simulink model "final_test"  (R2017a)
settings: Solver=VariableStepAuto  StartTime=0.0  StopTime=10.0  RelTol=1e-3
settings Model: Creator=ashwi  LastModifiedBy=ashwi

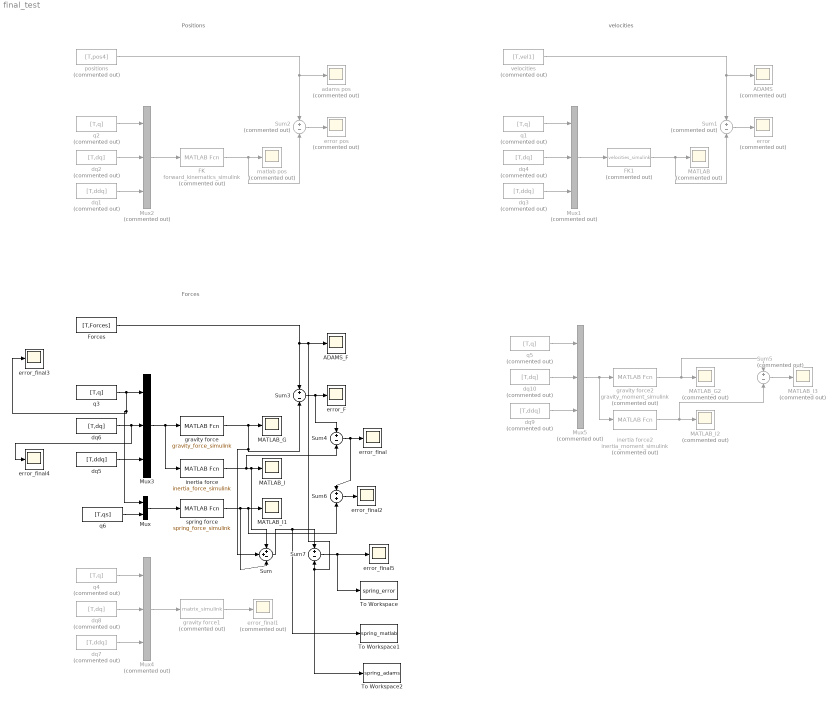
== system final_test ==
  note: Positions
  note: velocities
  note: Forces
  ADAMS : Scope  Commented=on
  ADAMS_F : Scope
  FK : MATLABFcn  Commented=on  MATLABFcn=forward_kinematics_simulink
  FK1 : MATLABFcn  Commented=on  MATLABFcn=velocities_simulink
  Forces : FromWorkspace  VariableName=[T,Forces]  SampleTime=0
  MATLAB : Scope  Commented=on
  MATLAB_G : Scope
  MATLAB_G2 : Scope  Commented=on
  MATLAB_I : Scope
  MATLAB_I1 : Scope
  MATLAB_I2 : Scope  Commented=on
  MATLAB_I3 : Scope  Commented=on
  Mux : Mux  Inputs=2
  Mux{1..2,4..5} (4 alike) : Mux  Commented=on  Inputs=3
  Mux3 : Mux  Inputs=3
  Sum : Sum  Inputs=++-
  Sum1 : Sum  Commented=on  Inputs=+-
  Sum2 : Sum  Commented=on  Inputs=+-
  Sum3 : Sum  Inputs=+-
  Sum4 : Sum  Inputs=+-
  Sum5 : Sum  Commented=on  Inputs=+-
  Sum6 : Sum
  Sum7 : Sum  Inputs=+-
  To Workspace : ToWorkspace  VariableName=spring_error  SaveFormat=Timeseries  SampleTime=-1
  To Workspace1 : ToWorkspace  VariableName=spring_matlab  SaveFormat=Timeseries  SampleTime=-1
  To Workspace2 : ToWorkspace  VariableName=spring_adams  SaveFormat=Timeseries  SampleTime=-1
  adams pos : Scope  Commented=on
  dq{1,3,7,9} (4 alike) : FromWorkspace  Commented=on  VariableName=[T,ddq]  SampleTime=0
  dq{2,4,8,10} (4 alike) : FromWorkspace  Commented=on  VariableName=[T,dq]  SampleTime=0
  dq5 : FromWorkspace  VariableName=[T,ddq]  SampleTime=0
  dq6 : FromWorkspace  VariableName=[T,dq]  SampleTime=0
  error : Scope  Commented=on
  error pos : Scope  Commented=on
  error_F : Scope
  error_final{,2..5} (5 alike) : Scope
  error_final1 : Scope  Commented=on
  gravity force : MATLABFcn  MATLABFcn=gravity_force_simulink
  gravity force1 : MATLABFcn  Commented=on  MATLABFcn=matrix_simulink
  gravity force2 : MATLABFcn  Commented=on  MATLABFcn=gravity_moment_simulink
  inertia force : MATLABFcn  MATLABFcn=inertia_force_simulink
  inertia force2 : MATLABFcn  Commented=on  MATLABFcn=inertia_moment_simulink
  matlab pos : Scope  Commented=on
  positions : FromWorkspace  Commented=on  VariableName=[T,pos4]  SampleTime=0
  q{1..2,4..5} (4 alike) : FromWorkspace  Commented=on  VariableName=[T,q]  SampleTime=0
  q3 : FromWorkspace  VariableName=[T,q]  SampleTime=0
  q6 : FromWorkspace  VariableName=[T,qs]  SampleTime=0
  spring force : MATLABFcn  MATLABFcn=spring_force_simulink
  velocities : FromWorkspace  Commented=on  VariableName=[T,vel1]  SampleTime=0
  wires:
  q2/1 -> Mux2/1
  positions/1 -> Sum2/1, adams pos/1
  Sum2/1 -> error pos/1
  dq2/1 -> Mux2/2
  dq1/1 -> Mux2/3
  Mux2/1 -> FK/1
  FK/1 -> Sum2/2, matlab pos/1
  velocities/1 -> Sum1/1, ADAMS/1
  FK1/1 -> Sum1/2, MATLAB/1
  Mux1/1 -> FK1/1
  q1/1 -> Mux1/1
  dq4/1 -> Mux1/2
  Sum1/1 -> error/1
  dq3/1 -> Mux1/3
  Forces/1 -> Sum3/1, To Workspace2/1, Sum7/2, ADAMS_F/1
  gravity force/1 -> Sum/2, Sum3/2, MATLAB_G/1
  Mux3/1 -> inertia force/1, gravity force/1
  q3/1 -> Mux/1, error_final3/1, Mux3/1
  dq6/1 -> error_final4/1, Mux3/2
  Sum3/1 -> Sum4/1, error_F/1
  dq5/1 -> Mux3/3
  inertia force/1 -> Sum4/2, Sum/1, MATLAB_I/1
  Sum4/1 -> Sum6/1, error_final/1
  gravity force1/1 -> error_final1/1
  Mux4/1 -> gravity force1/1
  dq7/1 -> Mux4/3
  q4/1 -> Mux4/1
  dq8/1 -> Mux4/2
  inertia force2/1 -> Sum5/2, MATLAB_I2/1
  q5/1 -> Mux5/1
  gravity force2/1 -> Sum5/1, MATLAB_G2/1
  dq9/1 -> Mux5/3
  Mux5/1 -> inertia force2/1, gravity force2/1
  dq10/1 -> Mux5/2
  Sum5/1 -> MATLAB_I3/1
  spring force/1 -> Sum/3, Sum6/2, MATLAB_I1/1
  Sum6/1 -> error_final2/1
  Sum/1 -> To Workspace1/1, Sum7/1
  Sum7/1 -> To Workspace/1, error_final5/1
  q6/1 -> Mux/2
  Mux/1 -> spring force/1
